simulink model "lab4_prep"  (R2023b)
settings: Solver=VariableStepAuto  StartTime=0.0  StopTime=10.0  RelTol=1e-10  AbsTol=1e-10
values from neighbouring files (symbols this model uses):
  Actrl = A - B*K - L*C    [lab4.m]
  Bctrl = [L B*K]    [lab4.m]
  C = [1 0 0 0; 0 0 1 0]    [lab4.m]
  Cctrl = -K    [lab4.m]
  Dctrl = [zeros(1,2) K]    [lab4.m]
  K = place(A, B, p_K)    [lab4.m]
  Ulim = 5.875    [lab4.m]
  x0 = [0; 0; pi/24; 0]    [lab4.m]
settings Model: Creator=Alfred  LastModifiedBy=markzhuang
settings SolverCC: AlgebraicLoopSolver=TrustRegion
settings DebuggingCC: UnconnectedInputMsg=warning  UnconnectedOutputMsg=warning  UnconnectedLineMsg=warning
settings ModelReferenceCC: EnableRefExpFcnMdlSchedulingChecks=on

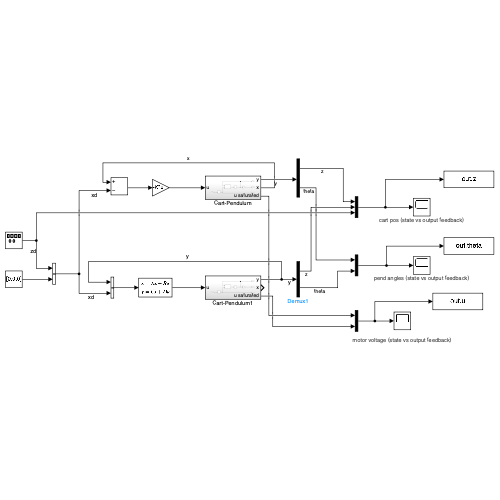
[thumbnail: Simulink's stored preview of the top-level diagram]
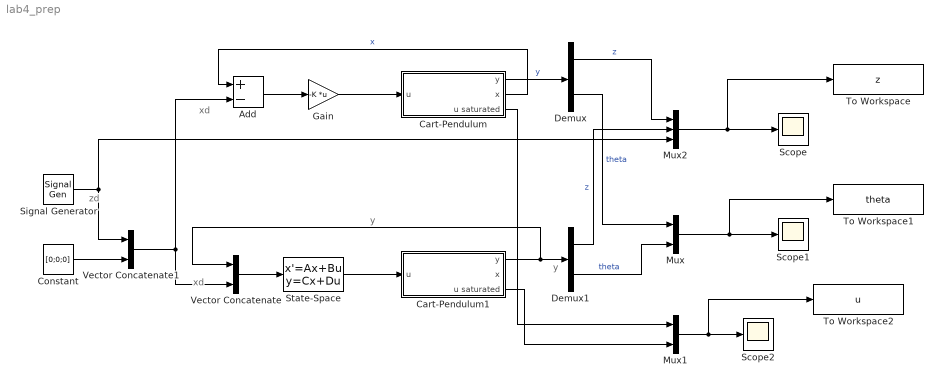
== system lab4_prep ==
  note: y
  note: y
  note: xd
  note: xd
  note: zd
  Add : Sum  Inputs=+-
  Cart-Pendulum : Subsystem
  Cart-Pendulum1 : Subsystem
  Constant : Constant  Value=[0;0;0]
  Demux : Demux  Outputs=2
  Demux1 : Demux  Outputs=2
  Gain : Gain  Gain=-K  Multiplication=Matrix(K*u)
  Mux : Mux  Inputs=2
  Mux1 : Mux  Inputs=2
  Mux2 : Mux  Inputs=3
  Scope : Scope
      settings: AttributesFormatString=cart pos (state vs output feedback)
  Scope1 : Scope
      settings: AttributesFormatString=pend angles (state vs output feedback)
  Scope2 : Scope
      settings: AttributesFormatString=motor voltage (state vs output feedback)
  Signal Generator : SignalGenerator  WaveForm=square  Amplitude=0.1  Frequency=0.1
  State-Space : StateSpace  A=Actrl  B=Bctrl  C=Cctrl  D=Dctrl  InitialCondition=x0
  To Workspace : ToWorkspace  VariableName=z  SaveFormat=Timeseries  SampleTime=-1
  To Workspace1 : ToWorkspace  VariableName=theta  SaveFormat=Timeseries  SampleTime=-1
  To Workspace2 : ToWorkspace  VariableName=u  SaveFormat=Timeseries  SampleTime=-1
  Vector Concatenate : Concatenate
  Vector Concatenate1 : Concatenate
  wires:
  Constant/1 -> Vector Concatenate1/2
  Signal Generator/1 -> Mux2/3, Vector Concatenate1/1
  Vector Concatenate1/1 -> Vector Concatenate/2, Add/2
  Vector Concatenate/1 -> State-Space/1
  State-Space/1 -> Cart-Pendulum1/1(u)
  Cart-Pendulum1/3(u saturated) -> Mux1/2
  Cart-Pendulum1/1(y) -> Demux1/1, Vector Concatenate/1
  Mux1/1 -> To Workspace2/1, Scope2/1
  Demux1/2 -> Mux/2  "theta"
  Mux/1 -> To Workspace1/1, Scope1/1
  Demux1/1 -> Mux2/2  "z"
  Add/1 -> Gain/1
  Gain/1 -> Cart-Pendulum/1(u)
  Cart-Pendulum/1(y) -> Demux/1  "y"
  Cart-Pendulum/2(x) -> Add/1  "x"
  Cart-Pendulum/3(u saturated) -> Mux1/1
  Demux/1 -> Mux2/1  "z"
  Demux/2 -> Mux/1  "theta"
  Mux2/1 -> To Workspace/1, Scope/1

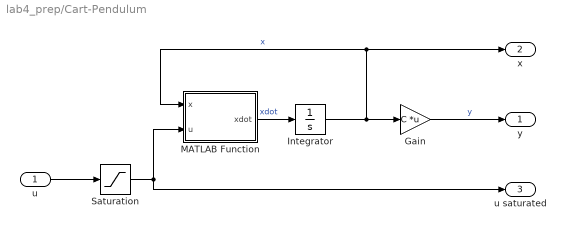
== system lab4_prep/Cart-Pendulum ==
  u : Inport
  Gain : Gain  Gain=C  Multiplication=Matrix(K*u)
  Integrator : Integrator  InitialCondition=x0
  MATLAB Function : MATLAB Function  TreatAsAtomicUnit=on
  Saturation : Saturate  UpperLimit=Ulim  LowerLimit=-Ulim
  y : Outport
  x : Outport  Port=2
  u saturated : Outport  Port=3
  wires:
  MATLAB Function/1(xdot) -> Integrator/1  "xdot"
  Integrator/1 -> MATLAB Function/1(x), x/1, Gain/1  "x"
  Gain/1 -> y/1  "y"
  u/1 -> Saturation/1
  Saturation/1 -> MATLAB Function/2(u), u saturated/1

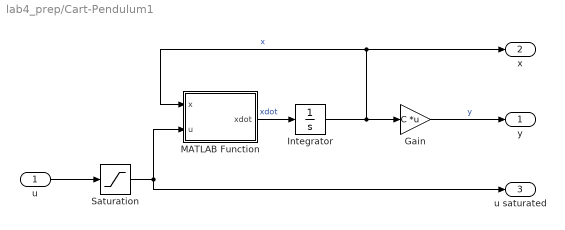
== system lab4_prep/Cart-Pendulum1 ==
  u : Inport
  Gain : Gain  Gain=C  Multiplication=Matrix(K*u)
  Integrator : Integrator  InitialCondition=x0
  MATLAB Function : MATLAB Function  TreatAsAtomicUnit=on
  Saturation : Saturate  UpperLimit=Ulim  LowerLimit=-Ulim
  y : Outport
  x : Outport  Port=2
  u saturated : Outport  Port=3
  wires:
  MATLAB Function/1(xdot) -> Integrator/1  "xdot"
  Integrator/1 -> MATLAB Function/1(x), x/1, Gain/1  "x"
  Gain/1 -> y/1  "y"
  u/1 -> Saturation/1
  Saturation/1 -> MATLAB Function/2(u), u saturated/1

== matlab function lab4_prep/Cart-Pendulum/MATLAB Function ==
  data: x input; u input; xdot output
function xdot = cartpend(x,u)

xdot = cartpend(x,u);

== matlab function lab4_prep/Cart-Pendulum1/MATLAB Function ==
  data: x input; u input; xdot output
function xdot = cartpend(x,u)

xdot = cartpend(x,u);
